simulink model "Task8"  (R2019b)
settings: Solver=VariableStepAuto  StartTime=0.0  StopTime=10.0  RelTol=1e-3
libraries: simulink x3, SignalEditorBlockLib x1
settings Model: Creator=12393  LastModifiedBy=12393

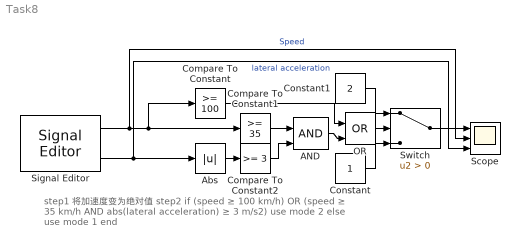
== system Task8 ==
  note: step1 将加速度变为绝对值
      | step2
      | if (speed ≥ 100 km/h) OR
      | (speed ≥ 35 km/h AND
      | abs(lateral acceleration) ≥ 3 m/s2)
      | use mode 2
      | else
      | use mode 1
      | end
  AND : Logic  IconShape=distinctive  AllPortsSameDT=off  OutDataTypeStr=boolean
  Abs : Abs
  Compare To Constant : simulink/Logic and Bit Operations/Compare To Constant  relop=>=  const=100  OutDataTypeStr=boolean
  Compare To Constant1 : simulink/Logic and Bit Operations/Compare To Constant  relop=>=  const=35  OutDataTypeStr=boolean
  Compare To Constant2 : simulink/Logic and Bit Operations/Compare To Constant  relop=>=  const=3  OutDataTypeStr=boolean
  Constant : Constant
  Constant1 : Constant  Value=2
  OR : Logic  Operator=OR  IconShape=distinctive  AllPortsSameDT=off  OutDataTypeStr=boolean
  Scope : Scope  NumInputPorts=3
  Signal Editor : SignalEditorBlockLib/Signal Editor  FileName=signal_Data.mat  ActiveScenario=data  ActiveSignal=speed  IsBus=off  OutputBusObjectStr=Bus: BusObject  SampleTime=0  Interpolate=off  ZeroCross=off  OutputAfterFinalValue=Setting to zero  Unit=inherit  PreserveSignalName=on
      settings: SourceProductName=Simulink
  Switch : Switch  Criteria=u2 > Threshold
  wires:
  Signal Editor/2 -> Scope/3, Abs/1  "lateral acceleration"
  Signal Editor/1 -> Scope/2, Compare To Constant/1, Compare To Constant1/1  "Speed"
  Abs/1 -> Compare To Constant2/1
  Compare To Constant1/1 -> AND/1
  Compare To Constant2/1 -> AND/2
  Compare To Constant/1 -> OR/1
  AND/1 -> OR/2
  OR/1 -> Switch/2
  Constant1/1 -> Switch/1
  Constant/1 -> Switch/3
  Switch/1 -> Scope/1
